simulink model "flexible_dipper_arm_kratos"  (R2020b)
settings: Solver=ode23t  StartTime=0.0  StopTime=10  RelTol=1e-3  AbsTol=1e-4  EnableMultiTasking=on
model workspace: external: MATLAB File sm_flexible_dipper_arm_parameters.m (data not in the file)
values from neighbouring files (symbols this model uses):
  arm = flexible_dipper_arm()    [main.m]
undefined symbols (not defined in the file or in its folder): base, common, cyl, floor, sigbuilder_block, tip, tower, wall, X, Y, Z
libraries: sm_lib x44, nesl_utility x11
(part 1 of 2)
Description:
  | Flexible Dipper Arm
settings Model: Creator=The MathWorks, Inc.  LastModifiedBy=sebastianadpr
settings SolverCC: AutoScaleAbsTol=off
settings DataIOCC: MaxDataPoints=10000  ReturnWorkspaceOutputs=off  SignalLoggingName=logsout_sm_flexible_dipper_arm
settings OptimizationCC: LifeSpan=inf
settings DebuggingCC: AllowSymbolicDim=off  SFUnexpectedBacktrackingDiag=warning  SFNoUnconditionalDefaultTransitionDiag=warning  SFExecutionAtInitializationDiag=none  ArithmeticOperatorsInVariantConditions=warning
settings SFSimCC: SimUseLocalCustomCode=off
settings RTWCC: RTWUseLocalCustomCode=off
settings CodeAppCC: StateflowObjectComments=on
settings GRTTargetCC: TargetLangStandard=C89/C90 (ANSI)
settings ConfigComp: CovMetricSettings=dw  CovSaveCumulativeToWorkspaceVar=on  CovSaveSingleToWorkspaceVar=on  CovExternalEMLEnable=off  CovSFcnEnable=off
settings SimscapeCC: SimscapeLogType=all  SimscapeLogSimulationStatistics=on  SimscapeLogName=simlog_sm_flexible_dipper_arm  SimscapeLogDataHistory=10000
settings ExplorerConfigSet: InternalSimMechanicsExplorerSettings="<ExplorerConfiguration><canonicalview>default</canonicalview><AnimationSetting><BasePlaybackSpeed>1.0</BasePlaybackSpeed><PlaybackSpeedFactor>1.0</PlaybackSpeedFactor></AnimationSetting><TilePanel><TileInfo><Tiles Columns=\"1\" Count=\"1\" Rows=\"1\"><Column Weight=\"1\"/><Row Weight=\"1\"/><Tile Height=\"1\" Width=\"1\" X=\"0\" Y=\"0\"/></Tiles></TileInfo><SceneInfo><SceneViewer><BGColor><R>0.60000002384185791</R><G>0.60000002384185791</G><B>0.60000002384185791</B></BGColor><Camera><DoPerspective>off</DoPerspective><Position><X>2.74170827827990626</X><Y>0.258291775228568943</Y><Z>1.76170825442195222</Z></Position><Center><X>1.32500002799872796</X><Y>1.67500002550974703</Y><Z>0.345000004140774086</Z></Center><Up><X>-0.408248290463863073</X><Y>0.408248290463863073</Y><Z>0.816496580927726145</Z></Up><ViewLimDist>1</ViewLimDist><YLim>1.74368889291546192</YLim><XLim>2.13533776534764597</XLim></Camera></SceneViewer></SceneInfo></TilePanel><MechEditorPanel><Cameras/><GfxPanelCameraMap/><VideoCreator><PlaybackSpeedRatio>1.0</PlaybackSpeedRatio><FrameRate>30</FrameRate><VideoFormat>Motion JPEG AVI</VideoFormat><FrameSize>auto</FrameSize></VideoCreator></MechEditorPanel></ExplorerConfiguration>"

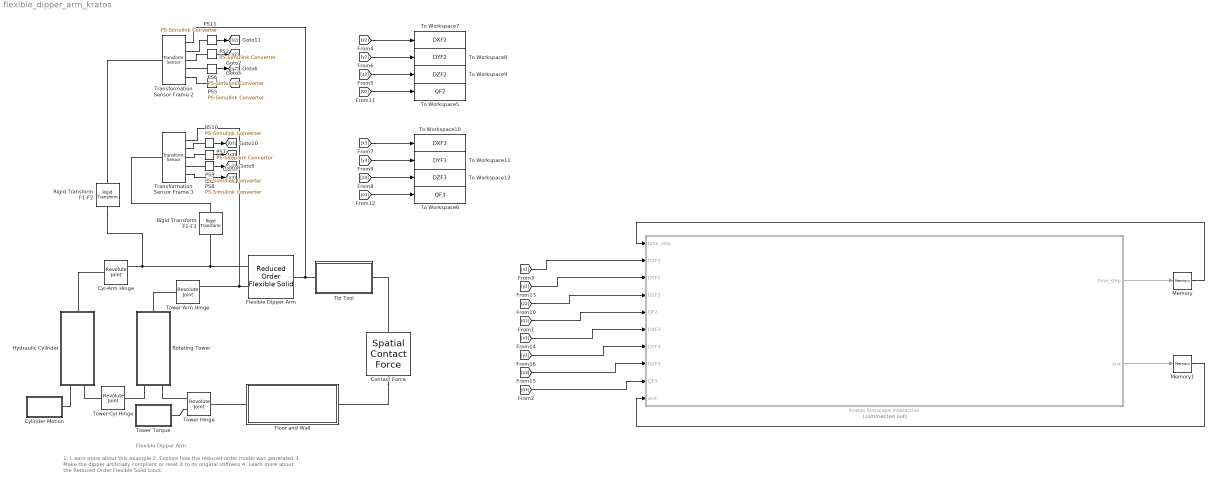
== system flexible_dipper_arm_kratos ==
  note: Flexible Dipper Arm
  note: 1. L earn more about this example
      | 2. Explore how the reduced-order model was generated
      | 3. Make the dipper artificially compliant or reset it to its original stiffness
      | 4. Learn more about the Reduced Order Flexible Solid block
  Contact Force : sm_lib/Forces and Torques/Spatial Contact Force  CoefficientOfDynamicFriction=contact.muk  CoefficientOfStaticFriction=contact.mus  NormalDamping=contact.c  NormalDampingUnits=N/(m/s)  NormalStiffness=contact.k  NormalStiffnessUnits=N/m  FrictionalCriticalVelocity=contact.vcr  FrictionalCriticalVelocityUnits=m/s  ZeroCrossDetectContactStartAndEnd=off  SenseFrictionalForceMagnitude=off  SenseNormalForceMagnitude=off  SenseSeparationDistance=off  NormalTransitionRegionWidth=contact.wtr  NormalTransitionRegionWidthUnits=m  FrictionType=SmoothStickSlip
  Cyl-Arm Hinge : sm_lib/Joints/Revolute Joint  JointMode=Normal  SenseConstraintForce=off  SenseConstraintForceX=off  SenseConstraintForceY=off  SenseConstraintForceZ=off  SenseConstraintTorque=off  SenseConstraintTorqueX=off  SenseConstraintTorqueY=off  SenseConstraintTorqueZ=off  SenseTotalForce=off  SenseTotalForceX=off  SenseTotalForceY=off  SenseTotalForceZ=off  SenseTotalTorque=off  SenseTotalTorqueX=off  SenseTotalTorqueY=off  SenseTotalTorqueZ=off  CompositeWrenchDir=FollowerOnBase  CompositeWrenchFrame=BaseFrame  EquilibriumPosition=0  EquilibriumPositionUnits=deg  SpringStiffness=0  SpringStiffnessUnits=N*m/deg  DampingCoefficient=0  DampingCoefficientUnits=N*m/(deg/s)  TorqueActuationMode=NoTorque  MotionActuationMode=ComputedMotion  SensePosition=on  SenseVelocity=off  SenseAcceleration=off  SenseTorqueForce=off  SenseLowerLimitTorqueForce=off  SenseUpperLimitTorqueForce=off  LowerLimitSpecify=off  LowerLimitBound=-90  LowerLimitBoundUnits=deg  LowerLimitStiffness=1e4  LowerLimitStiffnessUnits=N*m/deg  LowerLimitDamping=10  LowerLimitDampingUnits=N*m/(deg/s)  LowerLimitTransitionRegionWidth=0.1  LowerLimitTransitionRegionWidthUnits=deg  UpperLimitSpecify=off  UpperLimitBound=90  UpperLimitBoundUnits=deg  UpperLimitStiffness=1e4  UpperLimitStiffnessUnits=N*m/deg  UpperLimitDamping=10  UpperLimitDampingUnits=N*m/(deg/s)  UpperLimitTransitionRegionWidth=0.1  UpperLimitTransitionRegionWidthUnits=deg  PositionTargetSpecify=off  PositionTargetPriority=High  PositionTargetValue=0  PositionTargetValueUnits=deg  VelocityTargetSpecify=off  VelocityTargetPriority=High  VelocityTargetValue=0  VelocityTargetValueUnits=deg/s
      settings: SourceProductName=Multibody
  Cylinder Motion : Subsystem  mask(Cylinder actuation){p0=cyl.act.p0, a=cyl.act.a, T=cyl.act.T}
      mask prompts: p0 "Initial position (m)"; a "Position amplitude (m)"; T "Filtering constant (s)"
      mask help: Motion actuation profile for the cylinder that pushes the dipper up and down.
      mask DialogControl ActContainer Prompt: Actuation
      mask Display: image(fullfile(matlabroot,'toolbox','physmod','sm','smdemos','flexible_dipper_arm','images','sm_flexible_dipper_arm_CylinderActuation.png'));
  Flexible Dipper Arm : sm_lib/Body Elements/Flexible Bodies/Reduced Order Flexible Solid  GraphicAmbientColor=[0.15 0.15 0.15 1.0]  GraphicDiffuseColor=arm.c  DampingType=DampingMatrix  GraphicEmissiveColor=[0.0 0.0 0.0 1.0]  GeomFileName=sm_flexible_dipper_arm.step  GraphicType=PartitionedGeometry  MassMatrix=arm.M(1:18,1:18)  NumberOfInterfaceFrames=3  GraphicOpacity=arm.o  InterfaceFrameOrigins=arm.P  GraphicShininess=75  GraphicSpecularColor=[0.5 0.5 0.5 1.0]  StiffnessMatrix=arm.K(1:18,1:18)  GeomUnitType=FromFile  VisRecursionLimit=3  GraphicVisPropType=SimpleVisualProperties  LengthUnit=m  MassUnit=kg  TimeUnit=s  UnitSystemType=SI  ProportionalDampingAlpha=0  ProportionalDampingBeta=1e-4  UniformModalDampingRatio=0.01  DampingMatrix=arm.C(1:18,1:18)
      settings: SourceProductName=Multibody
  Floor and Wall : Subsystem  mask(Floor and Wall){wf=floor.w, tf=floor.t, cf=floor.c, of=floor.o, pb=base.p, hb=base.h, wb=base.w, cb=base.c, ob=base.o, pw=wall.p, hw=wall.h, ww=wall.w, tw=wall.t, cw=wall.c, ow=wall.o, dens=common.rho}
      mask prompts: wf "Width (m)"; tf "Thickness (m)"; cf "Color (RGB)"; of "Opacity (0-1)"; pb "Position (m)"; hb "Height (m)"; wb "Width (m)"; cb "Color (RGB)"; ob "Opacity (0-1)"; pw "Position (m)"; hw "Height (m)"; ww "Width (m)"; tw "Thickness (m)"; cw "Color (RGB)"; ow "Opacity (0-1)"; dens "Density (kg/m^3)"
      mask help: The floor supports a static base upon which the rotating tower is mounted, as well as a solid wall with which the tip of the arm will make contact to study the resulting vibrations.
      mask DialogControl FloorContainer Prompt: Floor
      mask DialogControl BaseContainer Prompt: Base
      mask DialogControl WallContainer Prompt: Wall
      mask DialogControl CommonContainer Prompt: Common properties
      mask Display: image(fullfile(matlabroot,'toolbox','physmod','sm','smdemos','flexible_dipper_arm','images','sm_flexible_dipper_arm_FloorAndWall.png'));
  Hydraulic Cylinder : Subsystem  mask(Hydraulic cylinder){ri=cyl.inner.r, ci=cyl.inner.c, oi=cyl.inner.o, Li=cyl.to_arm.L, Rhi=cyl.to_arm.r, Roi=cyl.to_arm.R, wi=cyl.to_arm.w, ro=cyl.outer.r, co=cyl.outer.c, oo=cyl.outer.o, Lo=cyl.to_base.L, Rho=cyl.to_base.r, to=cyl.to_base.t, wo=cyl.to_base.w, h=cyl.h, dens=common.rho}
      mask prompts: ri "Radius (m)"; ci "Color (RGB)"; oi "Opacity (0-1)"; Li "Length (m)"; Rhi "Hinge radius (m)"; Roi "Outer radius (m)"; wi "Width (m)"; ro "Radius (m)"; co "Color (RGB)"; oo "Opacity (0-1)"; Lo "Length (m)"; Rho "Hinge radius (m)"; to "Flange thickness (m)"; wo "Width (m)"; h "Cylinder length (m)"; dens "Density (kg/m^3)"
      mask help: The cylinder causes the dipper arm to rotate about the fulcrum point. It is driven by a prismatic motion input causing the tip of the dipper to move up and down.
      mask init:
      | theta1 = (-90:1:90)';
      | theta2 = (90:-1:-270)';
      | 
      | csi = [ 0                     ,  Roi              ; ...
      |         0                     , -Roi              ; ...
      |         Li + Roi*cosd(theta1) ,  Roi*sind(theta1) ; ...
      |         Li + Rhi*cosd(theta2) ,  Rhi*sind(theta2) ; ...
      |         Li                    ,  Roi              ];
      | 
      | cso = [ ri ,  h/2 ; ...
      |         ri , -h/2 ; ...
      |         ro , -h/2 ; ...
      |         ro ,  h/2 ];
      mask DialogControl InnerCylContainer Prompt: Inner cylinder
      mask DialogControl InnerAttContainer Prompt: Inner attachment
      mask DialogControl OuterCylContainer Prompt: Outer cylinder
      mask DialogControl OuterAttContainer Prompt: Outer attachment
      mask DialogControl CommonContainer Prompt: Common properties
      mask Display: image(fullfile(matlabroot,'toolbox','physmod','sm','smdemos','flexible_dipper_arm','images','sm_flexible_dipper_arm_Cylinder.png'));
  Kratos-Simscape interaction : MATLAB Function  Commented=on  TreatAsAtomicUnit=on
  Memory : Memory
  Memory1 : Memory  InitialCondition=-1
  PS{2,5..11} (8 alike) : nesl_utility/PS-Simulink Converter  PhysicalDomain=network_engine_domain  SubClassName=ps_output  LeftPortType=input  RightPortType=output  PseudoPeriodic=off  Frequencies=[]  Unit=mm  AffineConversion=off
      settings: SourceProductName=Utilities
  Rigid Transform F1-F2 : sm_lib/Frames and Transforms/Rigid Transform  TranslationMethod=Cartesian  TranslationStandardOffset=0  TranslationLengthUnit=m  TranslationStandardAxis=+Z  TranslationCartesianOffset="[-2  0  0]"  TranslationROffset=0  TranslationROffsetUnits=m  TranslationZOffset=0  TranslationZOffsetUnits=m  TranslationThetaOffset=0  TranslationThetaOffsetUnits=deg  RotationMethod=None  RotationAngleUnits=deg  RotationStandardAxis=+Z  RotationAngle=0.0  RotationArbitraryAxis=[0 0 1]  FollAlignAxisA=+X  BaseAlignAxisA=+Y  FollAlignAxisB=+Y  BaseAlignAxisB=+Z  RotationSequenceAxes=FollowerAxes  RotationSequence=XYX  RotationSequenceAngles=[0 0 0]  RotationSequenceAnglesUnits=deg  RotationMatrix=[1 0 0; 0 1 0; 0 0 1]
  Rigid Transform F1-F3 : sm_lib/Frames and Transforms/Rigid Transform  TranslationMethod=Cartesian  TranslationStandardOffset=0  TranslationLengthUnit=m  TranslationStandardAxis=+Z  TranslationCartesianOffset="[-0.5        0.13           0]"  TranslationROffset=0  TranslationROffsetUnits=m  TranslationZOffset=0  TranslationZOffsetUnits=m  TranslationThetaOffset=0  TranslationThetaOffsetUnits=deg  RotationMethod=None  RotationAngleUnits=deg  RotationStandardAxis=+Z  RotationAngle=0.0  RotationArbitraryAxis=[0 0 1]  FollAlignAxisA=+X  BaseAlignAxisA=+Y  FollAlignAxisB=+Y  BaseAlignAxisB=+Z  RotationSequenceAxes=FollowerAxes  RotationSequence=XYX  RotationSequenceAngles=[0 0 0]  RotationSequenceAnglesUnits=deg  RotationMatrix=[1 0 0; 0 1 0; 0 0 1]
  Rotating Tower : Subsystem  mask(Rotating Tower){ht=tower.h, wt=tower.w, tt=tower.t, hb=tower.base.h, wb=tower.base.w, La=tower.to_arm.L, Rha=tower.to_arm.r, Roa=tower.to_arm.R, wa=tower.to_arm.w, Lc=tower.to_cyl.L, Rhc=tower.to_cyl.r, Roc=tower.to_cyl.R, wc=tower.to_cyl.w, dens=common.rho, c=tower.c, o=tower.o}
      mask prompts: ht "Height (m)"; wt "Width (m)"; tt "Wall thickness (m)"; hb "Height (m)"; wb "Width (m)"; La "Length (m)"; Rha "Hinge radius (m)"; Roa "Outer radius (m)"; wa "Width (m)"; Lc "Length (m)"; Rhc "Hinge radius (m)"; Roc "Outer radius (m)"; wc "Width (m)"; dens "Density (kg/m^3)"; c "Color (RGB)"; o "Opacity (0-1)"
      mask help: The rotating tower supports the dipper arm and provides a connection point for the hydraulic cylinder as well. It is driven by a torque input that causes the dipper arm to rotate and "slap" the solid wall.
      mask init:
      | cst = [ -wt/2    , -wt/2    ; ...
      |          wt/2    , -wt/2    ; ...
      |          wt/2    ,  wt/2    ; ...
      |         -wt/2    ,  wt/2    ; ...
      |         -wt/2    , -wt/2    ; ...
      |         -wt/2+tt , -wt/2+tt ; ...
      |         -wt/2+tt ,  wt/2-tt ; ...
      |          wt/2-tt ,  wt/2-tt ; ...
      |          wt/2-tt , -wt/2+tt ; ...
      |         -wt/2+tt , -wt/2+tt ];
      | 
      | theta1 = (-90:1:90)';
      | theta2 = (90:-1:-270)';
      | 
      | csa = [ 0                     ,  Roa              ; ...
      |         0                     , -Roa              ; ...
      |         La + Roa*cosd(theta1) ,  Roa*sind(theta1) ; ...
      |         La + Rha*cosd(theta2) ,  Rha*sind(theta2) ; ...
      |         La                    ,  Roa              ];
      | 
      | csc = [ 0                     ,  Roc              ; ...
      |         0                     , -Roc              ; ...
      |         Lc + Roc*cosd(theta1) ,  Roc*sind(theta1) ; ...
      |         Lc + Rhc*cosd(theta2) ,  Rhc*sind(theta2) ; ...
      |         Lc                    ,  Roc              ];
      mask DialogControl TowerContainer Prompt: Tower
      mask DialogControl BaseContainer Prompt: Base
      mask DialogControl ArmContainer Prompt: Arm attachment
      mask DialogControl CylContainer Prompt: Cylinder attachment
      mask DialogControl CommonContainer Prompt: Common properties
      mask Display: image(fullfile(matlabroot,'toolbox','physmod','sm','smdemos','flexible_dipper_arm','images','sm_flexible_dipper_arm_Tower.png'));
  Tip Tool : Subsystem  mask(Tip Tool){Rb=tip.R, Rr=tip.r, L=tip.L, w=tip.w, t=tip.t, dens=common.rho, c=tip.c, o=tip.o}
      mask prompts: Rb "Radius (m)"; Rr "Radius (m)"; L "Length (m)"; w "Width (m)"; t "Thickness (m)"; dens "Density (kg/m^3)"; c "Color (RGB)"; o "Opacity (0-1)"
      mask help: The tip tool represents a part that can be attached at the end of the dipper arm to enable contact with a solid wall. It is made up of an attachment plate, a rod protruding from the plate and a solid ball attached at the end of the rod.
      mask DialogControl BallContainer Prompt: Ball
      mask DialogControl RodContainer Prompt: Rod
      mask DialogControl PlateContainer Prompt: Plate
      mask DialogControl CommonContainer Prompt: Common properties
      mask Display: image(fullfile(matlabroot,'toolbox','physmod','sm','smdemos','flexible_dipper_arm','images','sm_flexible_dipper_arm_TipTool.png'));
  To Workspace10 : ToWorkspace  VariableName=DXF3  SaveFormat=Timeseries  SampleTime=-1
  To Workspace11 : ToWorkspace  VariableName=DYF3  SaveFormat=Timeseries  SampleTime=-1
  To Workspace12 : ToWorkspace  VariableName=DZF3  SaveFormat=Timeseries  SampleTime=-1
  To Workspace5 : ToWorkspace  VariableName=QF2  SaveFormat=Timeseries  SampleTime=-1
  To Workspace6 : ToWorkspace  VariableName=QF3  SaveFormat=Timeseries  SampleTime=-1
  To Workspace7 : ToWorkspace  VariableName=DXF2  SaveFormat=Timeseries  SampleTime=-1
  To Workspace8 : ToWorkspace  VariableName=DYF2  SaveFormat=Timeseries  SampleTime=-1
  To Workspace9 : ToWorkspace  VariableName=DZF2  SaveFormat=Timeseries  SampleTime=-1
  Tower Hinge : sm_lib/Joints/Revolute Joint  JointMode=Normal  SenseConstraintForce=off  SenseConstraintForceX=off  SenseConstraintForceY=off  SenseConstraintForceZ=off  SenseConstraintTorque=off  SenseConstraintTorqueX=off  SenseConstraintTorqueY=off  SenseConstraintTorqueZ=off  SenseTotalForce=off  SenseTotalForceX=off  SenseTotalForceY=off  SenseTotalForceZ=off  SenseTotalTorque=off  SenseTotalTorqueX=off  SenseTotalTorqueY=off  SenseTotalTorqueZ=off  CompositeWrenchDir=FollowerOnBase  CompositeWrenchFrame=BaseFrame  EquilibriumPosition=0  EquilibriumPositionUnits=deg  SpringStiffness=0  SpringStiffnessUnits=N*m/deg  DampingCoefficient=tower.damping  DampingCoefficientUnits=N*m/(deg/s)  TorqueActuationMode=InputTorque  MotionActuationMode=ComputedMotion  SensePosition=off  SenseVelocity=off  SenseAcceleration=off  SenseTorqueForce=off  SenseLowerLimitTorqueForce=off  SenseUpperLimitTorqueForce=off  LowerLimitSpecify=off  LowerLimitBound=-90  LowerLimitBoundUnits=deg  LowerLimitStiffness=1e4  LowerLimitStiffnessUnits=N*m/deg  LowerLimitDamping=10  LowerLimitDampingUnits=N*m/(deg/s)  LowerLimitTransitionRegionWidth=0.1  LowerLimitTransitionRegionWidthUnits=deg  UpperLimitSpecify=off  UpperLimitBound=90  UpperLimitBoundUnits=deg  UpperLimitStiffness=1e4  UpperLimitStiffnessUnits=N*m/deg  UpperLimitDamping=10  UpperLimitDampingUnits=N*m/(deg/s)  UpperLimitTransitionRegionWidth=0.1  UpperLimitTransitionRegionWidthUnits=deg  PositionTargetSpecify=on  PositionTargetPriority=High  PositionTargetValue=45  PositionTargetValueUnits=deg  VelocityTargetSpecify=off  VelocityTargetPriority=High  VelocityTargetValue=0  VelocityTargetValueUnits=deg/s
      settings: SourceProductName=Multibody
  Tower Torque : Subsystem  mask(Tower actuation){t1=tower.act.t1, a1=tower.act.a1, t2=tower.act.t2, a2=tower.act.a2, t3=tower.act.t3, a3=tower.act.a3, t=tower.act.t}
      mask prompts: t1 "Step 1 time (s)"; a1 "Step 1 final value (nondim)"; t2 "Step 2 time (s)"; a2 "Step 2 final value (nondim)"; t3 "Step 3 time (s)"; a3 "Step 3 final value (nondim)"; t "Torque gain (N*m)"
      mask help: Torque actuation profile to rotate the dipper left and right.
      mask DialogControl ActContainer Prompt: Actuation
      mask Display: image(fullfile(matlabroot,'toolbox','physmod','sm','smdemos','flexible_dipper_arm','images','sm_flexible_dipper_arm_TowerActuation.png'));
  Tower-Arm Hinge : sm_lib/Joints/Revolute Joint  JointMode=Normal  SenseConstraintForce=on  SenseConstraintForceX=off  SenseConstraintForceY=off  SenseConstraintForceZ=off  SenseConstraintTorque=off  SenseConstraintTorqueX=off  SenseConstraintTorqueY=off  SenseConstraintTorqueZ=off  SenseTotalForce=off  SenseTotalForceX=off  SenseTotalForceY=off  SenseTotalForceZ=off  SenseTotalTorque=off  SenseTotalTorqueX=off  SenseTotalTorqueY=off  SenseTotalTorqueZ=off  CompositeWrenchDir=FollowerOnBase  CompositeWrenchFrame=BaseFrame  EquilibriumPosition=0  EquilibriumPositionUnits=deg  SpringStiffness=0  SpringStiffnessUnits=N*m/deg  DampingCoefficient=0  DampingCoefficientUnits=N*m/(deg/s)  TorqueActuationMode=NoTorque  MotionActuationMode=ComputedMotion  SensePosition=off  SenseVelocity=off  SenseAcceleration=off  SenseTorqueForce=off  SenseLowerLimitTorqueForce=off  SenseUpperLimitTorqueForce=off  LowerLimitSpecify=off  LowerLimitBound=-90  LowerLimitBoundUnits=deg  LowerLimitStiffness=1e4  LowerLimitStiffnessUnits=N*m/deg  LowerLimitDamping=10  LowerLimitDampingUnits=N*m/(deg/s)  LowerLimitTransitionRegionWidth=0.1  LowerLimitTransitionRegionWidthUnits=deg  UpperLimitSpecify=off  UpperLimitBound=90  UpperLimitBoundUnits=deg  UpperLimitStiffness=1e4  UpperLimitStiffnessUnits=N*m/deg  UpperLimitDamping=10  UpperLimitDampingUnits=N*m/(deg/s)  UpperLimitTransitionRegionWidth=0.1  UpperLimitTransitionRegionWidthUnits=deg  PositionTargetSpecify=on  PositionTargetPriority=Low  PositionTargetValue=0  PositionTargetValueUnits=deg  VelocityTargetSpecify=off  VelocityTargetPriority=High  VelocityTargetValue=0  VelocityTargetValueUnits=deg/s
      settings: SourceProductName=Multibody
  Tower-Cyl Hinge : sm_lib/Joints/Revolute Joint  JointMode=Normal  SenseConstraintForce=off  SenseConstraintForceX=off  SenseConstraintForceY=off  SenseConstraintForceZ=off  SenseConstraintTorque=off  SenseConstraintTorqueX=off  SenseConstraintTorqueY=off  SenseConstraintTorqueZ=off  SenseTotalForce=off  SenseTotalForceX=off  SenseTotalForceY=off  SenseTotalForceZ=off  SenseTotalTorque=off  SenseTotalTorqueX=off  SenseTotalTorqueY=off  SenseTotalTorqueZ=off  CompositeWrenchDir=FollowerOnBase  CompositeWrenchFrame=BaseFrame  EquilibriumPosition=0  EquilibriumPositionUnits=deg  SpringStiffness=0  SpringStiffnessUnits=N*m/deg  DampingCoefficient=0  DampingCoefficientUnits=N*m/(deg/s)  TorqueActuationMode=NoTorque  MotionActuationMode=ComputedMotion  SensePosition=off  SenseVelocity=off  SenseAcceleration=off  SenseTorqueForce=off  SenseLowerLimitTorqueForce=off  SenseUpperLimitTorqueForce=off  LowerLimitSpecify=off  LowerLimitBound=-90  LowerLimitBoundUnits=deg  LowerLimitStiffness=1e4  LowerLimitStiffnessUnits=N*m/deg  LowerLimitDamping=10  LowerLimitDampingUnits=N*m/(deg/s)  LowerLimitTransitionRegionWidth=0.1  LowerLimitTransitionRegionWidthUnits=deg  UpperLimitSpecify=off  UpperLimitBound=90  UpperLimitBoundUnits=deg  UpperLimitStiffness=1e4  UpperLimitStiffnessUnits=N*m/deg  UpperLimitDamping=10  UpperLimitDampingUnits=N*m/(deg/s)  UpperLimitTransitionRegionWidth=0.1  UpperLimitTransitionRegionWidthUnits=deg  PositionTargetSpecify=off  PositionTargetPriority=High  PositionTargetValue=0  PositionTargetValueUnits=deg  VelocityTargetSpecify=off  VelocityTargetPriority=High  VelocityTargetValue=0  VelocityTargetValueUnits=deg/s
      settings: SourceProductName=Multibody
  Transformation Sensor Frame 2 : sm_lib/Frames and Transforms/Transform Sensor  MeasurementFrame=NonRotatingFollower  SenseAngle=off  SenseAxis=off  SenseAngle1=off  SenseAngle2=off  SenseAngle3=off  SenseQ=on  SenseR=off  SenseOmegaX=off  SenseOmegaY=off  SenseOmegaZ=off  SenseOmega1=off  SenseOmega2=off  SenseOmega3=off  SenseQDot=off  SenseRDot=off  SenseAlphaX=off  SenseAlphaY=off  SenseAlphaZ=off  SenseAlpha1=off  SenseAlpha2=off  SenseAlpha3=off  SenseQDDot=off  SenseRDDot=off  SenseX=on  SenseY=on  SenseZ=on  SenseRad=off  SenseAzim=off  SenseDist=off  SenseInc=off  SenseXDot=off  SenseYDot=off  SenseZDot=off  SenseRadDot=off  SenseAzimDot=off  SenseDistDot=off  SenseIncDot=off  SenseXDDot=off  SenseYDDot=off  SenseZDDot=off  SenseRadDDot=off  SenseAzimDDot=off  SenseDistDDot=off  SenseIncDDot=off
      settings: SourceProductName=Multibody
  Transformation Sensor Frame 3 : sm_lib/Frames and Transforms/Transform Sensor  MeasurementFrame=NonRotatingFollower  SenseAngle=off  SenseAxis=off  SenseAngle1=off  SenseAngle2=off  SenseAngle3=off  SenseQ=on  SenseR=off  SenseOmegaX=off  SenseOmegaY=off  SenseOmegaZ=off  SenseOmega1=off  SenseOmega2=off  SenseOmega3=off  SenseQDot=off  SenseRDot=off  SenseAlphaX=off  SenseAlphaY=off  SenseAlphaZ=off  SenseAlpha1=off  SenseAlpha2=off  SenseAlpha3=off  SenseQDDot=off  SenseRDDot=off  SenseX=on  SenseY=on  SenseZ=on  SenseRad=off  SenseAzim=off  SenseDist=off  SenseInc=off  SenseXDot=off  SenseYDot=off  SenseZDot=off  SenseRadDot=off  SenseAzimDot=off  SenseDistDot=off  SenseIncDot=off  SenseXDDot=off  SenseYDDot=off  SenseZDDot=off  SenseRadDDot=off  SenseAzimDDot=off  SenseDistDDot=off  SenseIncDDot=off
      settings: SourceProductName=Multibody
  wires:
  PS6/1 -> [y2]
  PS2/1 -> [x2]
  PS5/1 -> [z2]
  PS9/1 -> [y3]
  PS7/1 -> [x3]
  PS8/1 -> [z3]
  [y2] -> To Workspace8/1
  [x2] -> To Workspace7/1
  [z2] -> To Workspace9/1
  [x3] -> To Workspace10/1
  [y3] -> To Workspace11/1
  [z3] -> To Workspace12/1
  PS10/1 -> [Q3]
  PS11/1 -> [Q2]
  [Q2] -> To Workspace5/1
  [Q3] -> To Workspace6/1
  [x2] -> Kratos-Simscape interaction/2(DXF2)
  [y2] -> Kratos-Simscape interaction/3(DYF2)
  [z2] -> Kratos-Simscape interaction/4(DZF2)
  [Q2] -> Kratos-Simscape interaction/5(QF2)
  [x3] -> Kratos-Simscape interaction/6(DXF3)
  [y3] -> Kratos-Simscape interaction/7(DYF3)
  [z3] -> Kratos-Simscape interaction/8(DZF3)
  [Q3] -> Kratos-Simscape interaction/9(QF3)
  Kratos-Simscape interaction/1(time_step) -> Memory/1
  Memory/1 -> Kratos-Simscape interaction/1("time_step ")
  Kratos-Simscape interaction/2(aux) -> Memory1/1
  Memory1/1 -> Kratos-Simscape interaction/10("aux ")
  connections:
  Flexible Dipper Arm/RConn1 -- Transformation Sensor Frame 2/RConn1 -- Tip Tool/LConn1
  Contact Force/LConn1 -- Floor and Wall/RConn1
  Cyl-Arm Hinge/LConn1 -- Hydraulic Cylinder/RConn1
  Tower-Cyl Hinge/RConn1 -- Hydraulic Cylinder/LConn2
  Rotating Tower/LConn1 -- Tower-Cyl Hinge/LConn1
  Flexible Dipper Arm/LConn2 -- Tower-Arm Hinge/RConn1 -- Transformation Sensor Frame 3/RConn1
  Cylinder Motion/RConn1 -- Hydraulic Cylinder/LConn1
  Tower Torque/RConn1 -- Tower Hinge/LConn2
  Transformation Sensor Frame 2/RConn4 -- PS6/LConn1
  PS2/LConn1 -- Transformation Sensor Frame 2/RConn3
  Transformation Sensor Frame 2/RConn5 -- PS5/LConn1
  Transformation Sensor Frame 3/RConn4 -- PS9/LConn1
  PS7/LConn1 -- Transformation Sensor Frame 3/RConn3
  Transformation Sensor Frame 3/RConn5 -- PS8/LConn1
  Tower-Arm Hinge/LConn1 -- Rotating Tower/RConn1
  PS10/LConn1 -- Transformation Sensor Frame 3/RConn2
  Transformation Sensor Frame 2/RConn2 -- PS11/LConn1
  Tower Hinge/LConn1 -- Rotating Tower/LConn2
  Tower Hinge/RConn1 -- Floor and Wall/LConn1
  Flexible Dipper Arm/LConn1 -- Rigid Transform F1-F2/RConn1 -- Cyl-Arm Hinge/RConn1 -- Rigid Transform F1-F3/RConn1
  Transformation Sensor Frame 3/LConn1 -- Rigid Transform F1-F3/LConn1
  Transformation Sensor Frame 2/LConn1 -- Rigid Transform F1-F2/LConn1
  Contact Force/RConn1 -- Tip Tool/RConn1

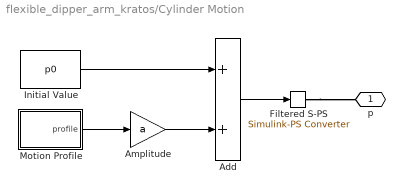
== system flexible_dipper_arm_kratos/Cylinder Motion ==
  Add : Sum
  Amplitude : Gain  Gain=a
  Filtered S-PS : nesl_utility/Simulink-PS Converter  PhysicalDomain=network_engine_domain  SubClassName=ps_input  LeftPortType=input  RightPortType=output  PseudoPeriodic=off  Frequencies=[]  NoiseDistribution=none  NoiseParameters=[]  Unit=m  AffineConversion=off  FilteringAndDerivatives=filter  SimscapeFilterOrder=2  InputFilterTimeConstant=T  UdotUserProvided=0
      settings: SourceProductName=Utilities
  Initial Value : Constant  Value=p0
  Motion Profile : Subsystem  Tag=STV Subsys  LoadFcn=sigbuilder_block('load');  StartFcn=sigbuilder_block('start');  StopFcn=sigbuilder_block('stop');  ClipboardFcn=sigbuilder_block('clipboard');  mask(Sigbuilder block){tuvar=[0:10]}
      mask help: Simulink:masks:SigbuilderBlock_MD
      mask init:
      | if ~strcmp(get_param(bdroot(gcbh),'SimulationStatus'),'stopped') tuvar = sigbuilder_block('maskInit'); end
      settings: CopyFcn=sigbuilder_block('copy');  DeleteFcn=sigbuilder_block('delete');  ModelCloseFcn=sigbuilder_block('modelClose');  PreSaveFcn=sigbuilder_block('preSave');  PauseFcn=sigbuilder_block('pause');  ContinueFcn=sigbuilder_block('continue');  NameChangeFcn=sigbuilder_block('namechange');  OpenFcn=sigbuilder_block('open',[220.941 114.641 550.787 319.456 ]);  CloseFcn=sigbuilder_block('close');
      mask Display: plot(0, 0, 100, 100,[2, 2, 32, 32, 2], [68, 8, 8, 68, 68],[32, 2], [38, 38], [32, 19, 2],[53, 60, 44], [32, 17, 17, 2],[16, 16, 31, 31]);txt = getActiveGroup(gcbh);text(2, 100, txt,'verticalAlignment', 'top');
  p : PMIOPort  Side=Right
  wires:
  Initial Value/1 -> Add/1
  Motion Profile/1(profile) -> Amplitude/1
  Amplitude/1 -> Add/2
  Add/1 -> Filtered S-PS/1
  connections:
  Filtered S-PS/RConn1 -- p/RConn1

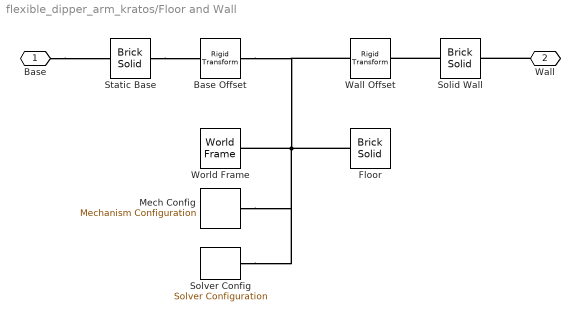
== system flexible_dipper_arm_kratos/Floor and Wall ==
  Base Offset : sm_lib/Frames and Transforms/Rigid Transform  TranslationMethod=Cartesian  TranslationStandardOffset=0  TranslationLengthUnit=m  TranslationStandardAxis=+Z  TranslationCartesianOffset=pb  TranslationROffset=0  TranslationROffsetUnits=m  TranslationZOffset=0  TranslationZOffsetUnits=m  TranslationThetaOffset=0  TranslationThetaOffsetUnits=deg  RotationMethod=None  RotationAngleUnits=deg  RotationStandardAxis=+Z  RotationAngle=0.0  RotationArbitraryAxis=[0 0 1]  FollAlignAxisA=+X  BaseAlignAxisA=+Y  FollAlignAxisB=+Y  BaseAlignAxisB=+Z  RotationSequenceAxes=FollowerAxes  RotationSequence=XYX  RotationSequenceAngles=[0 0 0]  RotationSequenceAnglesUnits=deg  RotationMatrix=[1 0 0; 0 1 0; 0 0 1]
      settings: SourceProductName=Multibody
  Floor : sm_lib/Body Elements/Brick Solid  GraphicAmbientColor=[0.15 0.15 0.15 1.0]  BasedOnType=Density  BrickDimensions=[wf wf tf]  BrickDimensionUnits=m  CenterOfMass=[0 0 0]  CenterOfMassUnits=m  GraphicDiffuseColor=cf  Density=dens  DensityUnits=kg/m^3  DoExposeReferenceFrame=off  GraphicEmissiveColor=[0.0 0.0 0.0 1.0]  ExportEntireGeometry=off  SerializedFrames=<Frames><Frame><Id>Frame1</Id><Value><Name>W</Name><Origin><Source>GeometricFeature</Source><FeatureName>-x -y +z point</FeatureName></Origin><PrimaryAxis><DefinedDirection>+Z</DefinedDirection><Source>ReferenceFrame</Source><SourceDirection>+Z</SourceDirection><FeatureName></FeatureName></PrimaryAxis><SecondaryAxis><DefinedDirection>+X</DefinedDirection><Source>ReferenceFrame</Source><SourceDirection>+X</SourceDirection><FeatureName></FeatureName></SecondaryAxis></Value></Frame></Frames>  MarkerShape=Sphere  MarkerSize=10  GraphicType=FromGeometry  InertiaType=CalculateFromGeometry  Mass=1  MassUnits=kg  MomentsOfInertia=[1 1 1]  MomentsOfInertiaUnits=kg*m^2  GraphicOpacity=of  ProductsOfInertia=[0 0 0]  ProductsOfInertiaUnits=kg*m^2  GraphicShininess=75  GraphicSpecularColor=[0.5 0.5 0.5 1.0]  GraphicVisPropType=SimpleVisualProperties
      settings: SourceProductName=Multibody
  Mech Config : sm_lib/Utilities/Mechanism Configuration  UniformGravity=None  GravityVector=[0 0 -9.80665]  GravityVectorUnits=m/s^2  GravityUnits=m/s^2  LinearizationDelta=0.001  JointModeTransitionNonlinearIterations=2
      settings: SourceProductName=Multibody
  Solid Wall : sm_lib/Body Elements/Brick Solid  GraphicAmbientColor=[0.15 0.15 0.15 1.0]  BasedOnType=Density  BrickDimensions=[tw ww hw]  BrickDimensionUnits=m  CenterOfMass=[0 0 0]  CenterOfMassUnits=m  GraphicDiffuseColor=cw  Density=dens  DensityUnits=kg/m^3  DoExposeReferenceFrame=off  GraphicEmissiveColor=[0.0 0.0 0.0 1.0]  ExportEntireGeometry=on  SerializedFrames=<Frames><Frame><Id>Frame1</Id><Value><Name>F</Name><Origin><Source>GeometricFeature</Source><FeatureName>-z surface</FeatureName></Origin><PrimaryAxis><DefinedDirection>+Z</DefinedDirection><Source>ReferenceFrame</Source><SourceDirection>+Z</SourceDirection><FeatureName></FeatureName></PrimaryAxis><SecondaryAxis><DefinedDirection>+X</DefinedDirection><Source>ReferenceFrame</Source><SourceDirection>+X</SourceDirection><FeatureName></FeatureName></SecondaryAxis></Value></Frame></Frames>  MarkerShape=Sphere  MarkerSize=10  GraphicType=FromGeometry  InertiaType=CalculateFromGeometry  Mass=1  MassUnits=kg  MomentsOfInertia=[1 1 1]  MomentsOfInertiaUnits=kg*m^2  GraphicOpacity=ow  ProductsOfInertia=[0 0 0]  ProductsOfInertiaUnits=kg*m^2  GraphicShininess=75  GraphicSpecularColor=[0.5 0.5 0.5 1.0]  GraphicVisPropType=SimpleVisualProperties
      settings: SourceProductName=Multibody
  Solver Config : nesl_utility/Solver Configuration  PhysicalDomain=network_engine_domain  SubClassName=solver  LeftPortType=input  RightPortType=generic  Tones=[]  Harmonics=[]  SimulateNoise=off  Profile=off  UseLocalSampling=off  EnableSwitchedLinearOptims=on  FrequencyDomain=off  UseCCode=off  RelTol=0.001  AbsTol=1e-06  MinStep=1e-09  ToWorkspace=off  RevertToSquareIcSolve=off  NumHomotopyIterations=100  PhasorMode=off  PhasorModeNumHarmonics=1  DoDC=off  ResidualTolerance=1e-09  UseLocalSolver=off  LocalSolverChoice=NE_BACKWARD_EULER_ADVANCER  LocalSolverSampleTime=0.001  DoFixedCost=off  MaxNonlinIter=3  MaxModeIter=2  ComputeImpulses=off  ImpulseIterations=1  LinearAlgebra=Sparse  EquationFormulation=NE_TIME_EF  DelaysMemoryBudget=1024  AutomaticFiltering=on  FilteringTimeConstant=0.001  PartitionStorageMethod=AS_NEEDED  PartitionMemoryBudget=1024  PartitionMethod=FAST
      settings: SourceProductName=Utilities
  Static Base : sm_lib/Body Elements/Brick Solid  GraphicAmbientColor=[0.15 0.15 0.15 1.0]  BasedOnType=Density  BrickDimensions=[wb wb hb]  BrickDimensionUnits=m  CenterOfMass=[0 0 0]  CenterOfMassUnits=m  GraphicDiffuseColor=cb  Density=dens  DensityUnits=kg/m^3  DoExposeReferenceFrame=off  GraphicEmissiveColor=[0.0 0.0 0.0 1.0]  ExportEntireGeometry=off  SerializedFrames=<Frames><Frame><Id>Frame1</Id><Value><Name>F</Name><Origin><Source>GeometricFeature</Source><FeatureName>-z surface</FeatureName></Origin><PrimaryAxis><DefinedDirection>+Z</DefinedDirection><Source>ReferenceFrame</Source><SourceDirection>+Z</SourceDirection><FeatureName></FeatureName></PrimaryAxis><SecondaryAxis><DefinedDirection>+X</DefinedDirection><Source>ReferenceFrame</Source><SourceDirection>+X</SourceDirection><FeatureName></FeatureName></SecondaryAxis></Value></Frame><Frame><Id>Frame2</Id><Value><Name>B</Name><Origin><Source>GeometricFeature</Source><FeatureName>+z surface</FeatureName></Origin><PrimaryAxis><DefinedDirection>+Z</DefinedDirection><Source>ReferenceFrame</Source><SourceDirection>+Z</SourceDirection><FeatureName></FeatureName></PrimaryAxis><SecondaryAxis><DefinedDirection>+X</DefinedDirection><Source>ReferenceFrame</Source><SourceDirection>+X</SourceDirection><FeatureName></FeatureName></SecondaryAxis></Value></Frame></Frames>  MarkerShape=Sphere  MarkerSize=10  GraphicType=FromGeometry  InertiaType=CalculateFromGeometry  Mass=1  MassUnits=kg  MomentsOfInertia=[1 1 1]  MomentsOfInertiaUnits=kg*m^2  GraphicOpacity=ob  ProductsOfInertia=[0 0 0]  ProductsOfInertiaUnits=kg*m^2  GraphicShininess=75  GraphicSpecularColor=[0.5 0.5 0.5 1.0]  GraphicVisPropType=SimpleVisualProperties
      settings: SourceProductName=Multibody
  Wall Offset : sm_lib/Frames and Transforms/Rigid Transform  TranslationMethod=Cartesian  TranslationStandardOffset=0  TranslationLengthUnit=m  TranslationStandardAxis=+Z  TranslationCartesianOffset=pw  TranslationROffset=0  TranslationROffsetUnits=m  TranslationZOffset=0  TranslationZOffsetUnits=m  TranslationThetaOffset=0  TranslationThetaOffsetUnits=deg  RotationMethod=None  RotationAngleUnits=deg  RotationStandardAxis=+Z  RotationAngle=30  RotationArbitraryAxis=[0 0 1]  FollAlignAxisA=+X  BaseAlignAxisA=+Y  FollAlignAxisB=+Y  BaseAlignAxisB=+Z  RotationSequenceAxes=FollowerAxes  RotationSequence=XYX  RotationSequenceAngles=[0 0 0]  RotationSequenceAnglesUnits=deg  RotationMatrix=[1 0 0; 0 1 0; 0 0 1]
      settings: SourceProductName=Multibody
  World Frame : sm_lib/Frames and Transforms/World Frame
      settings: SourceProductName=Multibody
  Base : PMIOPort  Side=Left
  Wall : PMIOPort  Port=2  Side=Right
  connections:
  Base/RConn1 -- Static Base/RConn1
  Wall Offset/LConn1 -- Base Offset/LConn1 -- World Frame/RConn1 -- Mech Config/RConn1 -- Solver Config/RConn1 -- Floor/LConn1
  Solid Wall/LConn1 -- Wall Offset/RConn1
  Wall/RConn1 -- Solid Wall/RConn1
  Static Base/LConn1 -- Base Offset/RConn1
